simulink model "Lab_01_PID"  (R2022b)
settings: Solver=FixedStepAuto  StartTime=0.0  StopTime=20  FixedStep=0.001  RelTol=1e-3
values from neighbouring files (symbols this model uses):
  degs2rpm = 0.166666666667    [parameters.mat]
  der =     [parameters.mat]
  sens =     [parameters.mat]
  Ts = 0.001    [parameters.mat]
undefined symbols (not defined in the file or in its folder): awu, DiscIntNeverNeededParam, National_Instruments, PCI, pid, simul
libraries: sldrtlib x3, simulink x1
settings Model: SimulationMode=external  ExtModeTrigDuration=50001  ExtModeTrigDurationFloating=50001  Creator=perondavid  LastModifiedBy=david
settings DataIOCC: LoggingToFile=on
settings HardwareCC: ProdBitPerLong=64  ProdHWDeviceType=Intel->x86-64 (Linux 64)
settings RTWCC: Description=Simulink Desktop Real-Time  SystemTargetFile=sldrt.tlc  TemplateMakefile=sldrt.tmf  RTWCompilerOptimization=on
settings CodeAppCC: MaxIdLength=95
settings SimulinkDesktopRealTimeCC: TargetLibSuffix=_sldrt.a  TargetPreCompLibLocation=C:\Program Files\MATLAB\R2022b\toolbox\sldrt\lib\win64

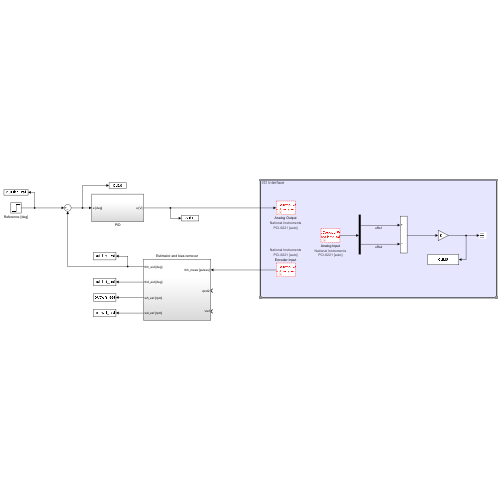
[thumbnail: Simulink's stored preview of the top-level diagram]
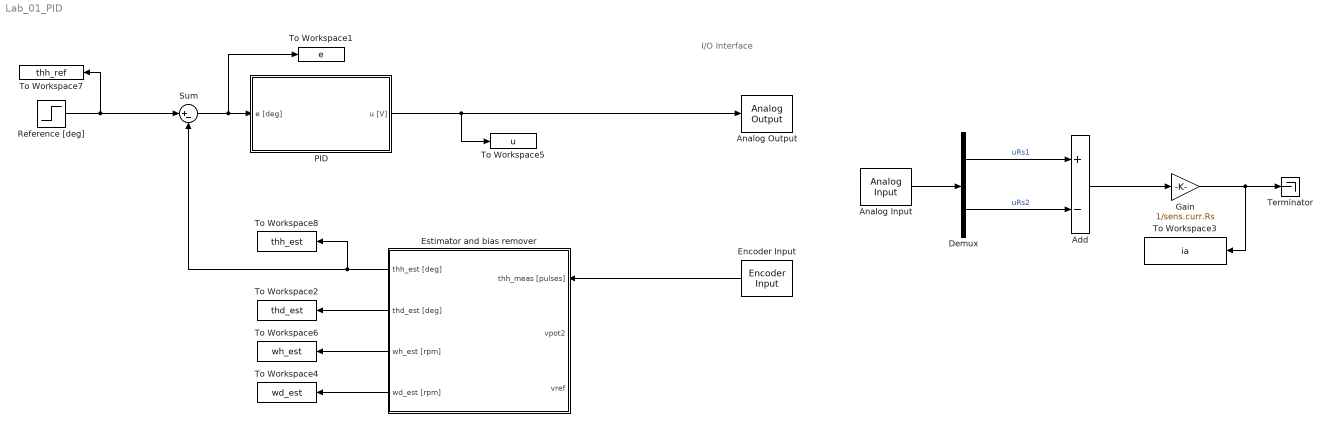
== system Lab_01_PID ==
  note: I/O Interface
  Add : Sum  Inputs=+-
  Analog Input : sldrtlib/Analog Input  SampleTime=-1  MaxMissedTicks=10  ShowMissedTicks=off  YieldWhenWaiting=off  DrvName=National_Instruments/PCI-6221  DrvAddress=4294967295  DrvOptions=[0 0 0 2 0]  Channels=[1, 2]  RangeMode=1  VoltRange=1  DataType=1
      settings: AttributesFormatString=National Instruments\nPCI-6221 [auto]
  Analog Output : sldrtlib/Analog Output  SampleTime=-1  MaxMissedTicks=10  ShowMissedTicks=off  YieldWhenWaiting=off  DrvName=National_Instruments/PCI-6221  DrvAddress=4294967295  DrvOptions=[0 0 0 2 0]  Channels=1  RangeMode=1  VoltRange=1  InitialValue=0  FinalValue=0
      settings: AttributesFormatString=National Instruments\nPCI-6221 [auto]
  Demux : Demux  Outputs=2
  Encoder Input : sldrtlib/Encoder Input  SampleTime=-1  MaxMissedTicks=10  ShowMissedTicks=off  YieldWhenWaiting=off  DrvName=National_Instruments/PCI-6221  DrvAddress=4294967295  DrvOptions=[0 0 0 2 0]  Channels=1  QuadMode=3  IndexPulse=1  InputFilter=Inf  DataType=1
      settings: AttributesFormatString=National Instruments\nPCI-6221 [auto]
  Estimator and bias remover : Subsystem
  Gain : Gain  Gain=1/sens.curr.Rs
  PID : Subsystem
  Reference [deg] : Step  After=simul.stepdeg  SampleTime=Ts
  Sum : Sum  Inputs=|+-
  Terminator : Terminator
  To Workspace1 : ToWorkspace  VariableName=e  SaveFormat=Structure With Time  SampleTime=-1
  To Workspace2 : ToWorkspace  VariableName=thd_est  SaveFormat=Structure With Time  SampleTime=Ts
  To Workspace3 : ToWorkspace  VariableName=ia  SaveFormat=Structure With Time  SampleTime=Ts
  To Workspace4 : ToWorkspace  VariableName=wd_est  SaveFormat=Structure With Time  SampleTime=Ts
  To Workspace5 : ToWorkspace  VariableName=u  SaveFormat=Structure With Time  SampleTime=Ts
  To Workspace6 : ToWorkspace  VariableName=wh_est  SaveFormat=Structure With Time  SampleTime=Ts
  To Workspace7 : ToWorkspace  VariableName=thh_ref  SaveFormat=Structure With Time  SampleTime=-1
  To Workspace8 : ToWorkspace  VariableName=thh_est  SaveFormat=Structure With Time  SampleTime=Ts
  wires:
  Demux/1 -> Add/1  "uRs1"
  Demux/2 -> Add/2  "uRs2"
  Add/1 -> Gain/1
  Gain/1 -> To Workspace3/1, Terminator/1
  Analog Input/1 -> Demux/1
  Sum/1 -> To Workspace1/1, PID/1(e [deg])
  Estimator and bias remover/2(thd_est [deg]) -> To Workspace2/1
  Estimator and bias remover/1(thh_est [deg]) -> To Workspace8/1, Sum/2
  Reference [deg]/1 -> To Workspace7/1, Sum/1
  Estimator and bias remover/3(wh_est [rpm]) -> To Workspace6/1
  Estimator and bias remover/4(wd_est [rpm]) -> To Workspace4/1
  PID/1(u [V]) -> Analog Output/1, To Workspace5/1
  Encoder Input/1 -> Estimator and bias remover/1(thh_meas [pulses])

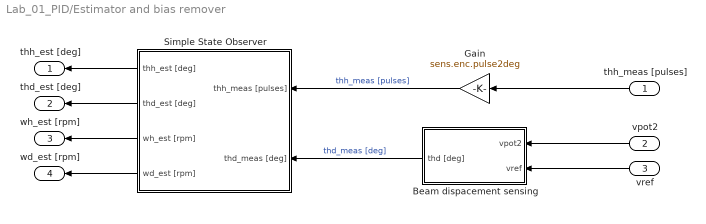
== system Lab_01_PID/Estimator and bias remover ==
  thh_meas [pulses] : Inport
  vpot2 : Inport  Port=2
  vref : Inport  Port=3
  Beam dispacement sensing : Subsystem
  Gain : Gain  Gain=sens.enc.pulse2deg
  Simple State Observer : Subsystem
  thh_est [deg] : Outport
  thd_est [deg] : Outport  Port=2
  wh_est [rpm] : Outport  Port=3
  wd_est [rpm] : Outport  Port=4
  wires:
  vpot2/1 -> Beam dispacement sensing/1(vpot2)
  vref/1 -> Beam dispacement sensing/2(vref)
  thh_meas [pulses]/1 -> Gain/1
  Gain/1 -> Simple State Observer/1(thh_meas [pulses])  "thh_meas [pulses]"
  Beam dispacement sensing/1(thd [deg]) -> Simple State Observer/2(thd_meas [deg])  "thd_meas [deg]"
  Simple State Observer/1(thh_est [deg]) -> thh_est [deg]/1
  Simple State Observer/2(thd_est [deg]) -> thd_est [deg]/1
  Simple State Observer/3(wh_est [rpm]) -> wh_est [rpm]/1
  Simple State Observer/4(wd_est [rpm]) -> wd_est [rpm]/1

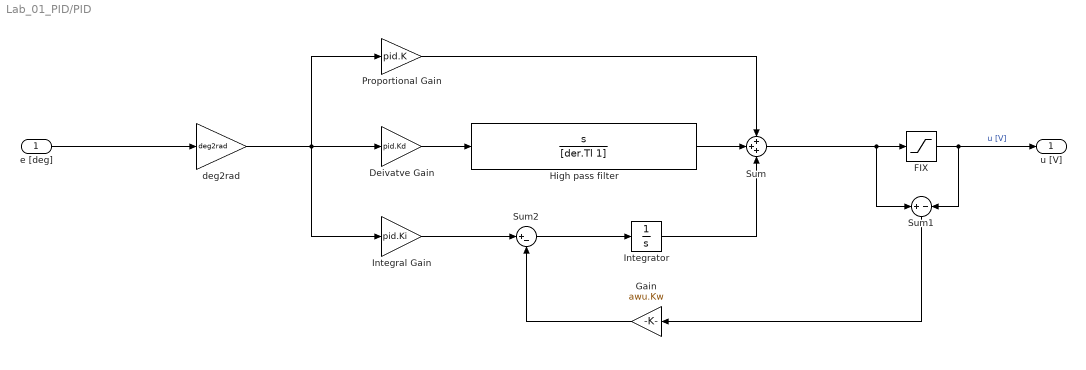
== system Lab_01_PID/PID ==
  e [deg] : Inport
  Deivatve Gain : Gain  Gain=pid.Kd
  "FIX " : Saturate  UpperLimit=10  LowerLimit=-10
  Gain : Gain  Gain=awu.Kw
  High pass filter : TransferFcn  Numerator=[1 0]  Denominator=[der.Tl 1]
  Integral Gain : Gain  Gain=pid.Ki
  Integrator : Integrator
  Proportional Gain : Gain  Gain=pid.K
  Sum : Sum  Inputs=+++
  Sum1 : Sum  Inputs=+-
  Sum2 : Sum  Inputs=|+-
  deg2rad : Gain  Gain=deg2rad
  u [V] : Outport
  wires:
  Deivatve Gain/1 -> High pass filter/1
  e [deg]/1 -> deg2rad/1
  "FIX "/1 -> Sum1/2, u [V]/1  "u [V]"
  deg2rad/1 -> Integral Gain/1, Deivatve Gain/1, Proportional Gain/1
  Proportional Gain/1 -> Sum/1
  Sum/1 -> Sum1/1, "FIX "/1
  High pass filter/1 -> Sum/2
  Integrator/1 -> Sum/3
  Integral Gain/1 -> Sum2/1
  Sum2/1 -> Integrator/1
  Gain/1 -> Sum2/2
  Sum1/1 -> Gain/1

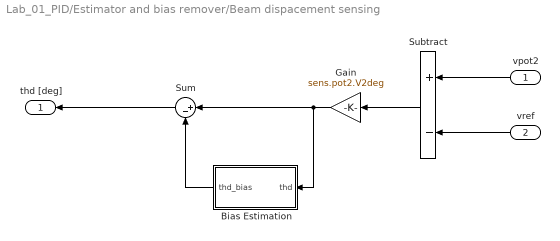
== system Lab_01_PID/Estimator and bias remover/Beam dispacement sensing ==
  vpot2 : Inport
  vref : Inport  Port=2
  Bias Estimation : Subsystem
  Gain : Gain  Gain=sens.pot2.V2deg
  Subtract : Sum  Inputs=+-
  Sum : Sum  Inputs=|+-
  thd [deg] : Outport
  wires:
  vref/1 -> Subtract/2
  vpot2/1 -> Subtract/1
  Subtract/1 -> Gain/1
  Gain/1 -> Sum/1, Bias Estimation/1(thd)
  Sum/1 -> thd [deg]/1
  Bias Estimation/1(thd_bias) -> Sum/2

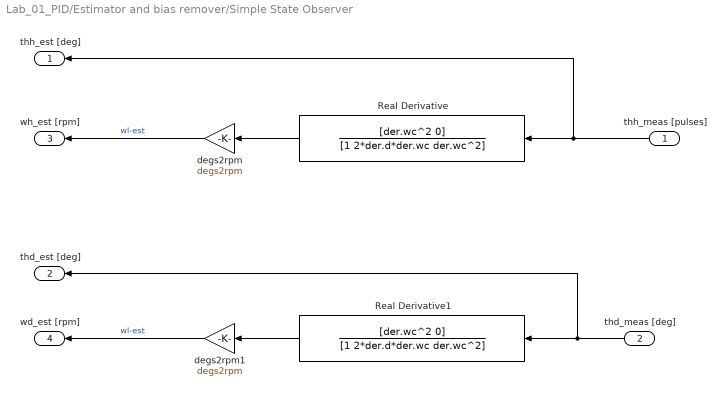
== system Lab_01_PID/Estimator and bias remover/Simple State Observer ==
  thh_meas [pulses] : Inport
  thd_meas [deg] : Inport  Port=2
  Real Derivative : TransferFcn  Numerator=[der.wc^2 0]  Denominator=[1 2*der.d*der.wc der.wc^2]
  Real Derivative1 : TransferFcn  Numerator=[der.wc^2 0]  Denominator=[1 2*der.d*der.wc der.wc^2]
  degs2rpm : Gain  Gain=degs2rpm
  degs2rpm1 : Gain  Gain=degs2rpm
  thh_est [deg] : Outport
  thd_est [deg] : Outport  Port=2
  wh_est [rpm] : Outport  Port=3
  wd_est [rpm] : Outport  Port=4
  wires:
  thd_meas [deg]/1 -> thd_est [deg]/1, Real Derivative1/1
  degs2rpm1/1 -> wd_est [rpm]/1  "wl-est"
  Real Derivative1/1 -> degs2rpm1/1
  degs2rpm/1 -> wh_est [rpm]/1  "wl-est"
  Real Derivative/1 -> degs2rpm/1
  thh_meas [pulses]/1 -> thh_est [deg]/1, Real Derivative/1

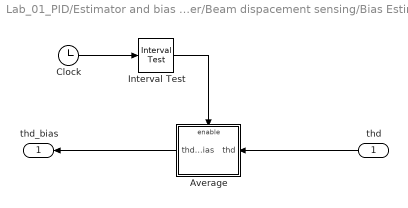
== system Lab_01_PID/Estimator and bias remover/Beam dispacement sensing/Bias Estimation ==
  thd : Inport
  Average : Subsystem
  Clock : Clock
  Interval Test : simulink/Logic and Bit Operations/Interval Test  IntervalClosedRight=on  uplimit=0.7  IntervalClosedLeft=on  lowlimit=0.2  OutDataTypeStr=boolean
  thd_bias : Outport
  wires:
  thd/1 -> Average/1(thd)
  Average/1(thd_bias) -> thd_bias/1
  Clock/1 -> Interval Test/1
  Interval Test/1 -> Average/Enable

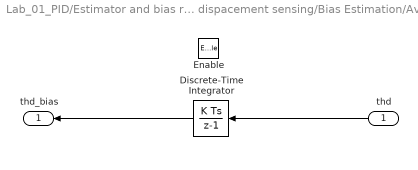
== system Lab_01_PID/Estimator and bias remover/Beam dispacement sensing/Bias Estimation/Average ==
  thd : Inport
  Enable : EnablePort
  Discrete-Time Integrator : DiscreteIntegrator  gainval=1/(0.7-0.2)  SampleTime=Ts  ICPrevOutput=DiscIntNeverNeededParam  ICPrevScaledInput=DiscIntNeverNeededParam
  thd_bias : Outport
  wires:
  thd/1 -> Discrete-Time Integrator/1
  Discrete-Time Integrator/1 -> thd_bias/1
